simulink model "C172_Plant_Controller2"  (R2025b)
settings: Solver=ode4  StartTime=0  StopTime=30  FixedStep=0.01  RelTol=1e-3
undefined symbols (not defined in the file): alt_target, C172MasterModel, df_deg_in, ki_alt, ki_v, kp_alt, kp_p, kp_phi, kp_v, kq, Ve_target
libraries: aerolibasang x2
settings Model: Creator=avi  LastModifiedBy=johns
settings DataIOCC: ExternalInput=thrust, df_deg, da_rad, de_rad, dr_rad  SaveFormat=StructureWithTime

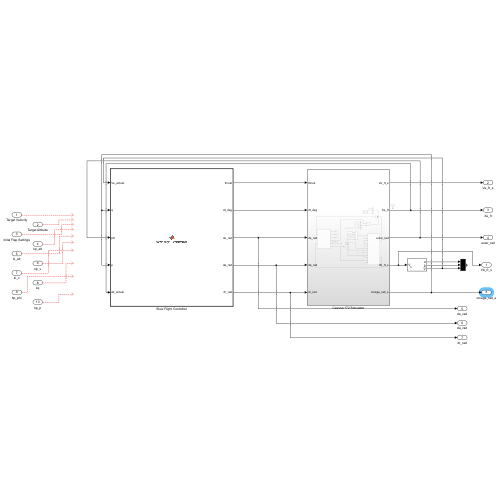
[thumbnail: Simulink's stored preview of the top-level diagram]
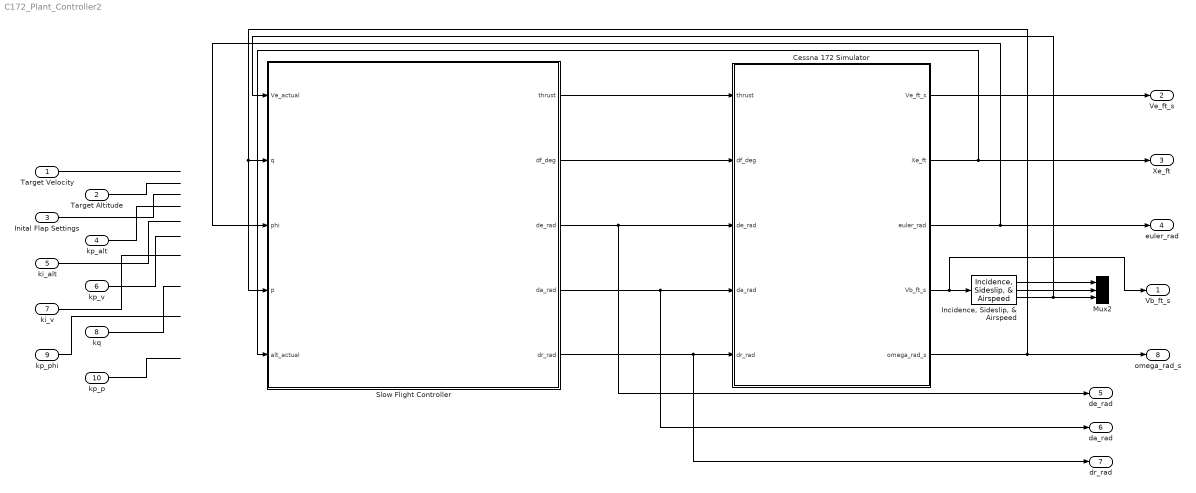
== system C172_Plant_Controller2 ==
  Target Velocity : Inport
  Target Altitude : Inport  Port=2
  Inital Flap Settings : Inport  Port=3
  kp_alt : Inport  Port=4
  ki_alt : Inport  Port=5
  kp_v : Inport  Port=6
  ki_v : Inport  Port=7
  kq : Inport  Port=8
  kp_phi : Inport  Port=9
  kp_p : Inport  Port=10
  Cessna 172 Simulator : Subsystem
  "Incidence, Sideslip, & Airspeed" : aerolibasang/Incidence, Sideslip, & Airspeed
  Mux2 : Mux  Inputs=3
  Slow Flight Controller : MATLAB Function  TreatAsAtomicUnit=on
  Vb_ft_s : Outport
  Ve_ft_s : Outport  Port=2
  Xe_ft : Outport  Port=3
  euler_rad : Outport  Port=4
  de_rad : Outport  Port=5
  da_rad : Outport  Port=6
  dr_rad : Outport  Port=7
  omega_rad_s : Outport  Port=8
  wires:
  Target Altitude/1 -> ?
  Target Velocity/1 -> ?
  Slow Flight Controller/2(df_deg) -> Cessna 172 Simulator/2(df_deg)
  Slow Flight Controller/1(thrust) -> Cessna 172 Simulator/1(thrust)
  Inital Flap Settings/1 -> ?
  kp_alt/1 -> ?
  kq/1 -> ?
  ki_v/1 -> ?
  kp_v/1 -> ?
  ki_alt/1 -> ?
  Slow Flight Controller/3(de_rad) -> Cessna 172 Simulator/3(de_rad), de_rad/1
  Slow Flight Controller/5(dr_rad) -> Cessna 172 Simulator/5(dr_rad), dr_rad/1
  Slow Flight Controller/4(da_rad) -> Cessna 172 Simulator/4(da_rad), da_rad/1
  kp_p/1 -> ?
  kp_phi/1 -> ?
  Cessna 172 Simulator/3(euler_rad) -> Slow Flight Controller/3(phi), euler_rad/1
  Cessna 172 Simulator/2(Xe_ft) -> Slow Flight Controller/5(alt_actual), Xe_ft/1
  Cessna 172 Simulator/1(Ve_ft_s) -> Ve_ft_s/1
  Cessna 172 Simulator/5(omega_rad_s) -> Slow Flight Controller/4(p), Slow Flight Controller/2(q), omega_rad_s/1
  Cessna 172 Simulator/4(Vb_ft_s) -> Vb_ft_s/1, "Incidence, Sideslip, & Airspeed"/1
  "Incidence, Sideslip, & Airspeed"/3 -> Slow Flight Controller/1(Ve_actual), Mux2/3
  "Incidence, Sideslip, & Airspeed"/2 -> Mux2/2
  "Incidence, Sideslip, & Airspeed"/1 -> Mux2/1

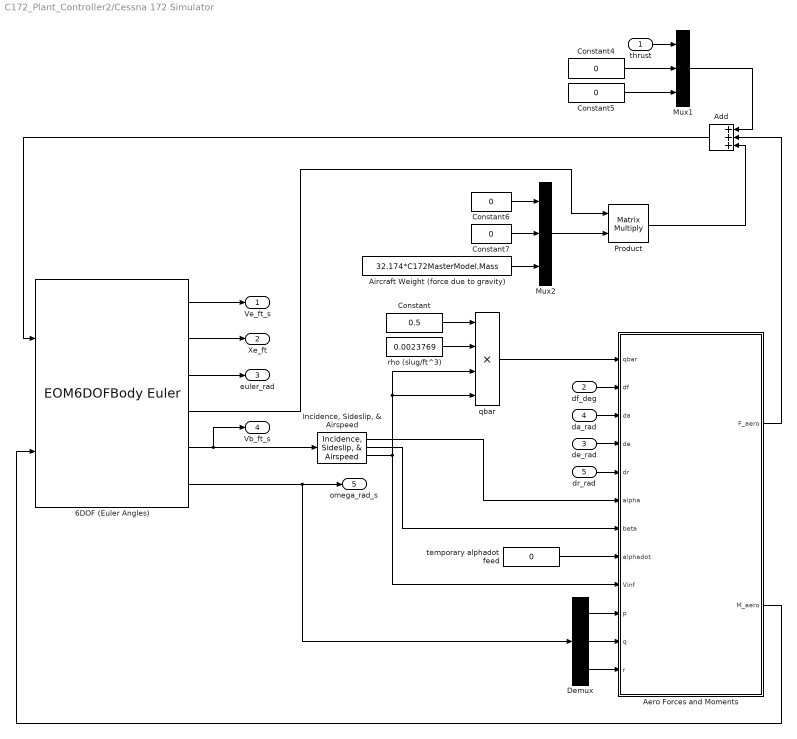
== system C172_Plant_Controller2/Cessna 172 Simulator ==
  thrust : Inport
  df_deg : Inport  Port=2
  de_rad : Inport  Port=3
  da_rad : Inport  Port=4
  dr_rad : Inport  Port=5
  6DOF (Euler Angles) : EOM6DOFBodyEuler  units=English (velocity in ft/s)  xme_0=Pos0  Vm_0=Vel0  eul_0=Att0  pm_0=Ome0  mass_0=C172MasterModel.Mass  inertia=C172MasterModel.Inertia
  Add : Sum  Inputs=+++
  Aero Forces and Moments : MATLAB Function  TreatAsAtomicUnit=on
  Aircraft Weight (force due to gravity) : Constant  Value=32.174*C172MasterModel.Mass
  Constant : Constant  Value=0.5
  Constant{4..7} (4 alike) : Constant  Value=0
  Demux : Demux  Outputs=3
  "Incidence, Sideslip, & Airspeed" : aerolibasang/Incidence, Sideslip, & Airspeed
  Mux1 : Mux  Inputs=3
  Mux2 : Mux  Inputs=3
  Product : Product  Multiplication=Matrix(*)
  qbar : Product  Inputs=4
  rho (slug/ft^3) : Constant  Value=0.0023769
  temporary alphadot feed : Constant  Value=0
  Ve_ft_s : Outport
  Xe_ft : Outport  Port=2
  euler_rad : Outport  Port=3
  Vb_ft_s : Outport  Port=4
  omega_rad_s : Outport  Port=5
  wires:
  temporary alphadot feed/1 -> Aero Forces and Moments/8(alphadot)
  "Incidence, Sideslip, & Airspeed"/2 -> Aero Forces and Moments/7(beta)
  Mux1/1 -> Add/1
  6DOF (Euler Angles)/1 -> Ve_ft_s/1
  df_deg/1 -> Aero Forces and Moments/2(df)
  rho (slug/ft^3)/1 -> qbar/2
  6DOF (Euler Angles)/4 -> Product/1
  Aero Forces and Moments/1(F_aero) -> Add/2
  Add/1 -> 6DOF (Euler Angles)/1
  "Incidence, Sideslip, & Airspeed"/3 -> Aero Forces and Moments/9(Vinf), qbar/4, qbar/3
  6DOF (Euler Angles)/5 -> Vb_ft_s/1, "Incidence, Sideslip, & Airspeed"/1
  de_rad/1 -> Aero Forces and Moments/4(de)
  qbar/1 -> Aero Forces and Moments/1(qbar)
  Constant6/1 -> Mux2/1
  "Incidence, Sideslip, & Airspeed"/1 -> Aero Forces and Moments/6(alpha)
  6DOF (Euler Angles)/2 -> Xe_ft/1
  dr_rad/1 -> Aero Forces and Moments/5(dr)
  Mux2/1 -> Product/2
  Demux/2 -> Aero Forces and Moments/11(q)
  Constant4/1 -> Mux1/2
  Demux/3 -> Aero Forces and Moments/12(r)
  da_rad/1 -> Aero Forces and Moments/3(da)
  Aero Forces and Moments/2(M_aero) -> 6DOF (Euler Angles)/2
  Constant7/1 -> Mux2/2
  6DOF (Euler Angles)/6 -> omega_rad_s/1, Demux/1
  Product/1 -> Add/3
  Constant5/1 -> Mux1/3
  Constant/1 -> qbar/1
  Aircraft Weight (force due to gravity)/1 -> Mux2/3
  6DOF (Euler Angles)/3 -> euler_rad/1
  thrust/1 -> Mux1/1
  Demux/1 -> Aero Forces and Moments/10(p)

== matlab function C172_Plant_Controller2/Slow Flight Controller ==
  settings: updateMethod=DISCRETE
  data: Ve_actual input; thrust output; df_deg output; de_rad output; q input; phi input; p input; alt_actual input; da_rad output; dr_rad output; Ve_target parameter; alt_target parameter; df_deg_in parameter; kp_alt parameter; ki_alt parameter; kp_v parameter; ki_v parameter; kq parameter; kp_phi parameter; kp_p parameter
function [thrust, df_deg, de_rad, da_rad, dr_rad] = slow_flight_controller(Ve_actual, q, phi, p, alt_actual, Ve_target, alt_target, df_deg_in, kp_alt, ki_alt, kp_v, ki_v, kq, kp_phi, kp_p)
    % --- INITIALIZATION ---
    persistent alt_int Ve_int
    if isempty(alt_int)
        alt_int = 0.0; 
        Ve_int = 0.0; 
    end
    dt = 0.01; 
    
    % --- 1. ROBUST STATE EXTRACTION ---
    % alt_actual(3) is Z-coord (Down). Must negate to get Altitude (Up).
    curr_alt = -double(alt_actual(3)); 
    curr_Ve  = double(Ve_actual(1));
    
    % Ensure we take the 1st element if these are vectors [phi; theta; psi]
    curr_phi = double(phi(1)); 
    curr_p   = double(p(1));
    curr_q   = double(q(2)); % If q is already pitch rate, q(1) is safe.

    % --- 2. ALTITUDE (Thrust) ---
    alt_err = double(alt_target) - curr_alt;
    alt_int = alt_int + (alt_err * dt);
    alt_int = max(min(alt_int, 500), -500); % Anti-windup
    
    thrust  = (kp_alt * alt_err) + (ki_alt * alt_int);
    thrust  = max(min(thrust, 2400), 0); 

    % --- 3. AIRSPEED (Elevator) ---
    % In Slow Flight: Pitch DOWN to gain speed.
    ve_err = double(Ve_target) - curr_Ve; 
    Ve_int = Ve_int + (ve_err * dt);
    Ve_int = max(min(Ve_int, 10), -10);
    
    % de_rad > 0 is usually Nose Down. 
    % Note the sign on kq: usually -(kq * q) to damp motion.
    de_rad = (kp_v * ve_err) + (ki_v * Ve_int) - (kq * curr_q);
    de_rad = max(min(de_rad, 0.45), -0.45); 

    % --- 4. ROLL & FLAPS ---
    da_rad = -(kp_phi * curr_phi) - (kp_p * curr_p);
    da_rad = max(min(da_rad, 0.4), -0.4); 
    
    dr_rad = 0.0; 
    df_deg = double(df_deg_in); 
end

== matlab function C172_Plant_Controller2/Cessna 172 Simulator/Aero Forces and Moments ==
  data: F_aero output size=[3,1]; M_aero output size=[3,1]; qbar input; df input; da input; de input; dr input; alpha input; beta input; alphadot input; Vinf input; p input; q input; r input; C172MasterModel parameter
function [F_aero, M_aero] = aero_forces_moments(qbar, df, da, de, dr, alpha, beta, alphadot, Vinf, p, q, r, C172MasterModel)

%% Load constant parameters from the C172 Master Model
Sw = C172MasterModel.Sw;
Cbar = C172MasterModel.Cbar;
bw = C172MasterModel.bw;
CG = C172MasterModel.CG;
AeroRP = C172MasterModel.AeroRP;

%% Forces

% Calculate all the drag force components
CDo = qbar*Sw*0.027;
CDDf = qbar*Sw*interp1(C172MasterModel.Tables.CDDf.RowBP, C172MasterModel.Tables.CDDf.Data, df);
CDwbh = qbar*Sw*interp2(C172MasterModel.Tables.CDwbh.ColBP, C172MasterModel.Tables.CDwbh.RowBP, C172MasterModel.Tables.CDwbh.Data, df, alpha);
CDbeta = qbar*Sw*norm(beta)*0.15;
% Calculate total drag force
Drag = CDo + CDDf + CDwbh + CDbeta;

if isnan(CDDf)
    error('Simulation halted: CDDf lookup out of bounds. Input was %f.', df);
end
if isnan(CDwbh)
    error('Simulation halted: CDwbh lookup out of bounds. Input was %f and %f.', df, alpha);
end

% Calculate all the side force components
CYb = qbar*Sw*interp2(C172MasterModel.Tables.CYb.ColBP, C172MasterModel.Tables.CYb.RowBP, C172MasterModel.Tables.CYb.Data, df, beta);
CYdr = qbar*Sw*dr*0.15;
% Calculate total side force
Side = CYb + CYdr;

if isnan(CYb)
    error('Simulation halted: CYb lookup out of bounds. Input was %f and %f.', df, beta);
end

% Calculate all the lift force components
CLwbh = qbar*Sw*interp1(C172MasterModel.Tables.CLwbh.RowBP, C172MasterModel.Tables.CLwbh.Data, alpha);
CLDf = qbar*Sw*interp1(C172MasterModel.Tables.CLDf.RowBP, C172MasterModel.Tables.CLDf.Data, df);
CLDe = qbar*Sw*de*0.43;
CLadot = qbar*Sw*alphadot*(Cbar/(2*Vinf))*1.7;
CLq = qbar*Sw*q*(Cbar/(2*Vinf))*3.9;
% Calculate total lift force
Lift = CLwbh + CLDf + CLDe + CLadot + CLq;

if isnan(CLwbh)
    error('Simulation halted: CLwbh lookup out of bounds. Input was %f.', alpha);
end
if isnan(CLDf)
    error('Simulation halted: CLDf lookup out of bounds. Input was %f.', df);
end


%% Moments

% Calculate roll moment components
Clb = qbar*Sw*bw*beta*(-0.092);
Clp = qbar*Sw*bw*(bw/(2*Vinf))*p*(-0.484);
Clr = qbar*Sw*bw*(bw/(2*Vinf))*r*interp1(C172MasterModel.Tables.Clr.RowBP, C172MasterModel.Tables.Clr.Data, alpha);
ClDa = qbar*Sw*bw*da*0.2;
Cldr = qbar*Sw*bw*dr*0.0147;
% Calculate total roll moment
Roll = Clb + Clp + Clr + ClDa + Cldr;

if isnan(Clr)
    error('Simulation halted: Clr lookup out of bounds. Input was %f.', alpha);
end


% Calculate pitch moment components
Cmo = qbar*Sw*Cbar*interp1(C172MasterModel.Tables.Cmo.RowBP, C172MasterModel.Tables.Cmo.Data, qbar);
Cmalpha = qbar*Sw*Cbar*alpha*(-1);
Cmq = qbar*Sw*Cbar*(Cbar/(2*Vinf))*q*(-12.4);
Cmadot = qbar*Sw*Cbar*(Cbar/(2*Vinf))*alphadot*(-7.27);
Cmde = qbar*Sw*Cbar*de*(-1);
Cmdf = qbar*Sw*Cbar*interp1(C172MasterModel.Tables.Cmdf.RowBP, C172MasterModel.Tables.Cmdf.Data, df);
% Calculate total pitch moment
Pitch = Cmo + Cmalpha + Cmq + Cmadot + Cmde + Cmdf;

if isnan(Cmo)
    error('Simulation halted: Cmo lookup out of bounds. Input was %f.', qbar);
end
if isnan(Cmdf)
    error('Simulation halted: Cmdf lookup out of bounds. Input was %f.', df);
end


% Calculate yaw moment components
Cnb = qbar*Sw*bw*interp1(C172MasterModel.Tables.Cnb.RowBP, C172MasterModel.Tables.Cnb.Data, beta);
Cnr = qbar*Sw*bw*(bw/(2*Vinf))*r*(-0.0937);
Cnda = qbar*Sw*bw*da*interp2(C172MasterModel.Tables.Cnda.ColBP, C172MasterModel.Tables.Cnda.RowBP, C172MasterModel.Tables.Cnda.Data, beta, alpha);
Cnp = qbar*Sw*bw*(bw/(2*Vinf))*p*interp1(C172MasterModel.Tables.Cnp.RowBP, C172MasterModel.Tables.Cnp.Data, alpha);
Cndr = qbar*Sw*bw*dr*(-0.0645);
% Calculate total yaw moment
Yaw = Cnb + Cnr + Cnda + Cnp + Cndr;

if isnan(Cnb)
    error('Simulation halted: Cnb lookup out of bounds. Input was %f.', beta);
end
if isnan(Cnda)
    error('Simulation halted: Cnda lookup out of bounds. Input was %f and %f.', beta, alpha);
end
if isnan(Cnp)
    error('Simulation halted: Cnp lookup out of bounds. Input was %f.', alpha);
end



%% Transform Forces to Body Axes
% Lift and Drag rotated by alpha. Sideforce is already in Body Y.
F_Ax = -Drag * cos(alpha) + Lift * sin(alpha);
F_Ay = Side;
F_Az = -Drag * sin(alpha) - Lift * cos(alpha);

F_aero = [F_Ax; F_Ay; F_Az];

%% Map Structural Coordinates to Body Frame Moment Arms
% Structural: +X aft, +Y right, +Z up
% Body:       +X fwd, +Y right, +Z down
dx_struct = AeroRP(1) - CG(1);
dy_struct = AeroRP(2) - CG(2);
dz_struct = AeroRP(3) - CG(3);

rx = -dx_struct;
ry = dy_struct;
rz = -dz_struct;

%% Calculate Induced Moments at CG (Cross Product: r x F)
delta_Roll  = (ry * F_Az) - (rz * F_Ay);
delta_Pitch = (rz * F_Ax) - (rx * F_Az);
delta_Yaw   = (rx * F_Ay) - (ry * F_Ax);

%% Sum Total Moments in Body Axes
M_Total_Roll  = Roll + delta_Roll;
M_Total_Pitch = Pitch + delta_Pitch;
M_Total_Yaw   = Yaw + delta_Yaw;

M_aero = [M_Total_Roll; M_Total_Pitch; M_Total_Yaw];

end
